simulink model "nucleo_f446_lm75b"  (R2015a)
settings: Solver=FixedStepDiscrete  SolverMode=SingleTasking  StartTime=0.0  StopTime=10.0  FixedStep=1e-3  RelTol=1e-3
libraries: mbed_lib x3, mbed_i2c_sensors x1, mbed_targets_stm_nucleo_f446 x1
settings Model: CovSFcnEnable=off  Creator=oh  LastModifiedBy=oh
settings OptimizationCC: OptimizeModelRefInitCode=on  LifeSpan=1
settings DebuggingCC: SolverPrmCheckMsg=warning
settings HardwareCC: ProdLargestAtomicInteger=Long  ProdLargestAtomicFloat=Double  ProdEndianess=LittleEndian  ProdHWDeviceType=ARM Compatible->ARM Cortex
settings RTWCC: SystemTargetFile=mbed.tlc  TemplateMakefile=mbed.tmf  Description=Mbed Target (Embedded Target)  TargetLang=C++
settings CodeAppCC: IgnoreCustomStorageClasses=off
settings STFCustomTargetCC: CombineOutputUpdateFcns=on  SupportContinuousTime=off  SupportVariableSizeSignals=off  SystemTargetFile=mbed.tlc
settings ERTTargetCC: SupportContinuousTime=off  SupportVariableSizeSignals=off  ERTCustomFileTemplate=mbed_file_process.tlc

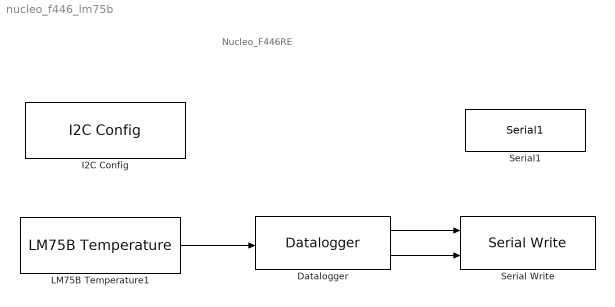
== system nucleo_f446_lm75b ==
  note: Nucleo_F446RE
  Datalogger : mbed_lib/Utilities/Datalogger  TypeInputPorts={ 'single' 1 }  TypeOfInputs={'1*single'}  BufferSize=100  errEn=off  SampleTime=-1
  I2C Config : mbed_lib/I2C/I2C Config  Priority=0  I2cPort=1  SParameter6=100000  SParameter2=B  SParameter3=9  SParameter4=B  SParameter5=8
  LM75B Temperature1 : mbed_i2c_sensors/LM75B Temperature  I2cPort=1  SampleTime=1
  Serial Write : mbed_lib/Serial/Serial Write  SerialPort=1  numData=on  SampleTime=-1
  Serial1 : mbed_targets_stm_nucleo_f446/Serial1  Parameter1=0  BaudRate=9600
  wires:
  LM75B Temperature1/1 -> Datalogger/1
  Datalogger/1 -> Serial Write/1
  Datalogger/2 -> Serial Write/2
